simulink model "SSC17_QuanserPart3_SetupSIMULINK_NL"  (R2016b)
settings: Solver=ode45  StartTime=0.0  StopTime=60  RelTol=1e-3  EnableMultiTasking=on
settings Model: Creator=am13440  LastModifiedBy=Alex
settings DataIOCC: SaveFormat=Array
settings OptimizationCC: LifeSpan=inf
settings DebuggingCC: UnderspecifiedInitializationDetection=Classic  MergeDetectMultiDrivingBlocksExec=none  SolverPrmCheckMsg=warning  StateNameClashWarn=warning  SFUnexpectedBacktrackingDiag=warning  SFNoUnconditionalDefaultTransitionDiag=warning  SFExecutionAtInitializationDiag=none
settings HardwareCC: ProdBitPerPointer=32  ProdBitPerSizeT=32  ProdBitPerPtrDiffT=32  ProdLargestAtomicFloat=None  ProdIntDivRoundTo=Undefined  ProdEndianess=Unspecified  ProdWordSize=32  ProdHWDeviceType=32-bit Generic
settings ModelReferenceCC: PropagateSignalLabelsOutOfModel=off
settings GRTTargetCC: TargetLangStandard=C89/C90 (ANSI)  GeneratePreprocessorConditionals=Disable all
settings ConfigComp: CovMetricSettings=dw  CovHtmlReporting=on  CovSaveCumulativeToWorkspaceVar=on  CovSaveSingleToWorkspaceVar=on  CovExternalEMLEnable=off  CovSFcnEnable=off

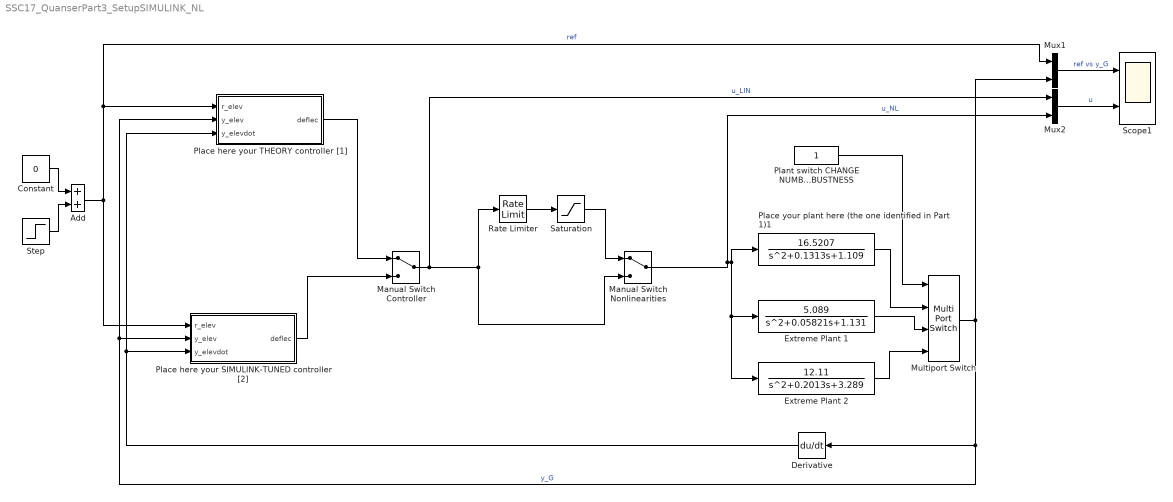
== system SSC17_QuanserPart3_SetupSIMULINK_NL ==
  Add : Sum
  Constant : Constant  Value=0
  Derivative : Derivative  CoefficientInTFapproximation=100
  Extreme Plant 1 : TransferFcn  Numerator=[5.089]  Denominator="[1  0.05821   1.131]"
  Extreme Plant 2 : TransferFcn  Numerator=[12.11]  Denominator="[1    0.2013   3.289]"
  Manual Switch Controller : ManualSwitch
  Manual Switch Nonlinearities : ManualSwitch
  Multiport Switch : MultiPortSwitch
  Mux1 : Mux  Inputs=2
  Mux2 : Mux  Inputs=2
  Place here your SIMULINK-TUNED controller [2] : Subsystem
  Place here your THEORY controller [1] : Subsystem
  Place your plant here (the one identified in Part 1)1 : TransferFcn  Numerator=[16.5207]  Denominator=[1 0.1313 1.109]
  Plant switch CHANGE NUMBER [1 / 2 /  3] TO SELECT AMONG PLANTS AND TEST ROBUSTNESS : Constant
  Rate Limiter : RateLimiter  RisingSlewLimit=3.5  FallingSlewLimit=-3.5  SampleTimeMode=inherited
  Saturation : Saturate  UpperLimit=0.4  LowerLimit=-0.4
  Scope1 : Scope  NumInputPorts=2
  Step : Step  Time=10  SampleTime=0
  wires:
  Constant/1 -> Add/1
  Step/1 -> Add/2
  Add/1 -> Place here your SIMULINK-TUNED controller [2]/1(r_elev), Place here your THEORY controller [1]/1(r_elev), Mux1/1  "ref"
  Derivative/1 -> Place here your SIMULINK-TUNED controller [2]/3(y_elevdot), Place here your THEORY controller [1]/3(y_elevdot)
  Manual Switch Nonlinearities/1 -> Mux2/2, Place your plant here (the one identified in Part 1)1/1, Extreme Plant 1/1, Extreme Plant 2/1  "u_NL"
  Place your plant here (the one identified in Part 1)1/1 -> Multiport Switch/2
  Extreme Plant 1/1 -> Multiport Switch/3
  Extreme Plant 2/1 -> Multiport Switch/4
  Plant switch CHANGE NUMBER [1 / 2 /  3] TO SELECT AMONG PLANTS AND TEST ROBUSTNESS/1 -> Multiport Switch/1
  Multiport Switch/1 -> Place here your SIMULINK-TUNED controller [2]/2(y_elev), Place here your THEORY controller [1]/2(y_elev), Derivative/1, Mux1/2  "y_G"
  Place here your THEORY controller [1]/1(deflec) -> Manual Switch Controller/1
  Place here your SIMULINK-TUNED controller [2]/1(deflec) -> Manual Switch Controller/2
  Rate Limiter/1 -> Saturation/1
  Manual Switch Controller/1 -> Mux2/1, Rate Limiter/1, Manual Switch Nonlinearities/2  "u_LIN"
  Saturation/1 -> Manual Switch Nonlinearities/1
  Mux1/1 -> Scope1/1  "ref vs y_G"
  Mux2/1 -> Scope1/2  "u"

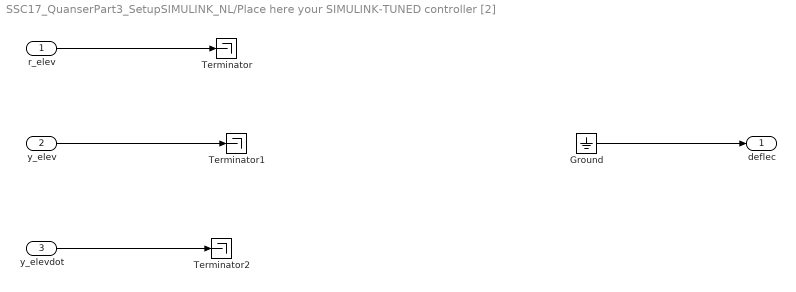
== system SSC17_QuanserPart3_SetupSIMULINK_NL/Place here your SIMULINK-TUNED controller [2] ==
  r_elev : Inport
  y_elev : Inport  Port=2
  y_elevdot : Inport  Port=3
  Ground : Ground
  Terminator : Terminator
  Terminator1 : Terminator
  Terminator2 : Terminator
  deflec : Outport
  wires:
  r_elev/1 -> Terminator/1
  y_elev/1 -> Terminator1/1
  y_elevdot/1 -> Terminator2/1
  Ground/1 -> deflec/1

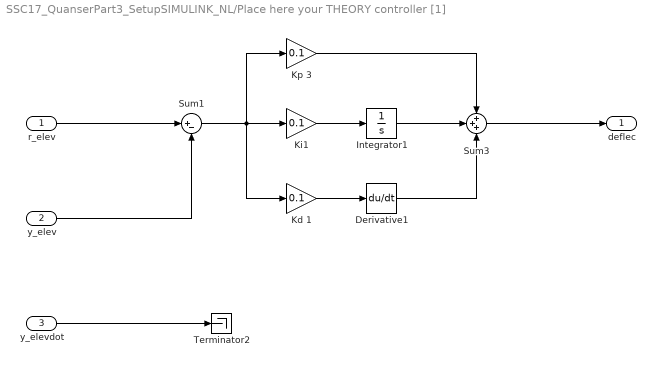
== system SSC17_QuanserPart3_SetupSIMULINK_NL/Place here your THEORY controller [1] ==
  r_elev : Inport
  y_elev : Inport  Port=2
  y_elevdot : Inport  Port=3
  Derivative1 : Derivative
  Integrator1 : Integrator
  Kd 1 : Gain  Gain=0.1
  Ki1 : Gain  Gain=0.1
  Kp 3 : Gain  Gain=0.1
  Sum1 : Sum  Inputs=|+-
  Sum3 : Sum  Inputs=+++
  Terminator2 : Terminator
  deflec : Outport
  wires:
  y_elevdot/1 -> Terminator2/1
  y_elev/1 -> Sum1/2
  r_elev/1 -> Sum1/1
  Sum1/1 -> Kp 3/1, Kd 1/1, Ki1/1
  Ki1/1 -> Integrator1/1
  Integrator1/1 -> Sum3/2
  Kd 1/1 -> Derivative1/1
  Derivative1/1 -> Sum3/3
  Kp 3/1 -> Sum3/1
  Sum3/1 -> deflec/1
